simulink model "blocks"  (R2024a)
settings: Solver=VariableStepAuto  StartTime=0.0  StopTime=100000  RelTol=1e-3  AbsTol=1e-3  EnableMultiTasking=on
PreLoadFcn:
  | LeadAcidBatteryWithDashboardBlocksINI;
values from neighbouring files (symbols this model uses):
  Kt = [0.80,1.10,1.20,1.12;]    [LeadAcidBatteryWithDashboardBlocksINI.m]
  Kt_Temps = [25 40 60 75]    [LeadAcidBatteryWithDashboardBlocksINI.m]
  theta_f = -40    [LeadAcidBatteryWithDashboardBlocksINI.m]
  theta_init = 25    [LeadAcidBatteryWithDashboardBlocksINI.m]
libraries: fl_lib x13, nesl_utility x7, LeadAcidBattery_lib x6, SignalEditorBlockLib x1
CloseFcn:
  | try,close(h1_LeadAcidBatteryWithDashboardBlocks),end
  | clear h1_LeadAcidBatteryWithDashboardBlocks
  | 
  | clear simlog_LeadAcidBatteryWithDashboardBlocks
Description:
  | Lead-Acid Battery with Dashboard Blocks
settings Model: PacingRate=2000  Creator=The MathWorks, Inc.  LastModifiedBy=owner's
settings SolverCC: AutoScaleAbsTol=off  AlgebraicLoopSolver=TrustRegion  MaxZcPerStep=1
settings DataIOCC: LimitDataPoints=on  MaxDataPoints=10000  SaveFormat=Array  ReturnWorkspaceOutputs=off
settings OptimizationCC: ReuseModelBlockBuffer=off  LifeSpan=inf
settings DebuggingCC: UnconnectedInputMsg=warning  UnconnectedOutputMsg=warning  UnconnectedLineMsg=warning  AllowSymbolicDim=off  PregeneratedLibrarySubsystemCodeDiagnostic=none  SFUnexpectedBacktrackingDiag=warning  SFNoUnconditionalDefaultTransitionDiag=warning  SFExecutionAtInitializationDiag=none  ArithmeticOperatorsInVariantConditions=warning
settings HardwareCC: ProdBitPerPointer=32  ProdBitPerSizeT=32  ProdBitPerPtrDiffT=32  ProdLargestAtomicFloat=None  ProdIntDivRoundTo=Undefined  ProdEndianess=Unspecified  ProdWordSize=32  ProdHWDeviceType=32-bit Generic
settings ModelReferenceCC: EnableRefExpFcnMdlSchedulingChecks=on  PropagateSignalLabelsOutOfModel=off
settings SFSimCC: SimUseLocalCustomCode=off  CustomCodeUndefinedFunction=UseInterfaceOnly
settings RTWCC: RTWUseLocalCustomCode=off  GPUComputeCapability=3.5  DLArmComputeVersion=19.05
settings CodeAppCC: StateflowObjectComments=on
settings GRTTargetCC: TargetLangStandard=C89/C90 (ANSI)
settings ConfigComp: CovMetricSettings=dw  CovSaveCumulativeToWorkspaceVar=on  CovSaveSingleToWorkspaceVar=on  CovExternalEMLEnable=off  CovSFcnEnable=off
settings SimscapeCC: SimscapeLogType=all  SimscapeLogSimulationStatistics=on  SimscapeLogToSDI=on  SimscapeLogName=simlog_LeadAcidBatteryWithDashboardBlocks  SimscapeLogDataHistory=10000

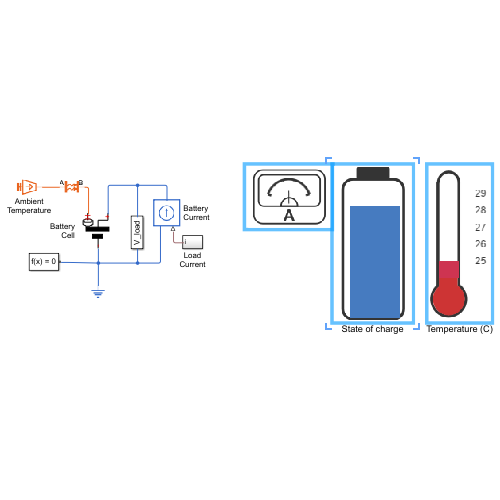
[thumbnail: Simulink's stored preview of the top-level diagram]
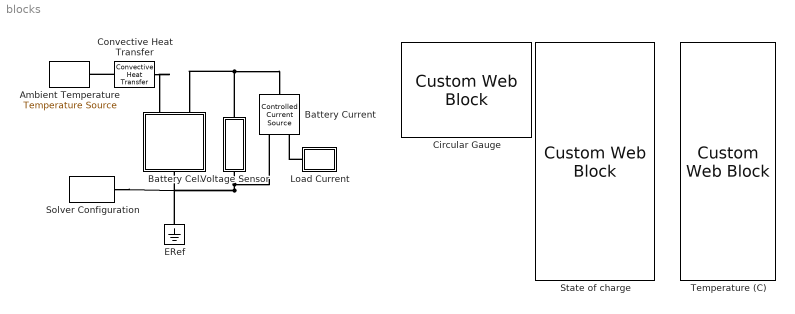
== system blocks ==
  Ambient Temperature : fl_lib/Thermal/Thermal Sources/Temperature Source  temperature=25 degC
  Battery Cell : Subsystem  Tag=PublishSubsystem
      mask Display:
      | % Battery icon
      | plot([0 0],[-1.5 -0.4])
      | plot([0 0 0.8 0.8],[0.2 0.9 0.9 1.5])
      | patch([-1 1 1 -1]*0.4,[1 1 -1 -1]*0.15-0.5,[0;0;0]);
      | patch([-1 1 1 -1]*0.9,[1 1 -1 -1]*0.15+0.1,[0;0;0]);
      | 
      | % Thermal port
      | plot([-1.2,-1.2],[0.5,0.9])
      | plot([-0.4,-0.4],[0.5,0.9])
      | plot([-0.8,-0.8],[0.9,1.5])
      | plot(0.35*cos(0:2*pi/50:2*pi)-0.8,0.15*sin(0:2*pi/50:2*pi)+0.85)
      | plot(0.35*cos(pi:2*pi/50:2*pi)-0.8,0.15*sin(pi:2*pi/50:2*pi)+0.55)
      | 
      | % Plot points to set plot range
      | color('white');plot(1.5,1.5);plot(-1.5,-1.5)
      | 
      | color('red')
      | port_label('LConn',1,'H')
      | port_label('LConn',2,'+')
      | port_label('RConn',1,'-')
  Battery Current : fl_lib/Electrical/Electrical Sources/Controlled Current Source
  Circular Gauge : CustomWebBlock  LabelPosition=Hide  ShowInitialText=on  Configuration="{\"components\":[{\"name\":\"CircularScaleComponent\",\"settings\":{\"bounds\":{\"max\":12,\"min\":-12,\"tickInterval\":23.9999999999999},\"direction\":\"cw\",\"flipLimits\":0,\"innerRadius\":0.75,\"internalTickHeightScaleFactor\":1,\"labelColor\":[38,38,38],\"labelFont\":{\"font\":\"Arial\",\"fontSize\":12},\"labelRadius\":0.528,\"labelTransparency\":0,\"minorTickHeightScaleFactor\":0.2,\"needleImage\":{\"size\":[96,288],\"src\":\"data:image\\/svg+xml;base64,PHN2ZyB3aWR0aD0iOTYiIGhlaWdodD0iMjg4IiB4bWxucz0iaHR0cDovL3d3dy53My5vcmcvMjAwMC9zdmciIHhtbG5zOnhsaW5rPSJodHRwOi8vd3d3LnczLm9yZy8xOTk5L3hsaW5rIiBvdmVyZmxvdz0iaGlkZGVuIj48ZGVmcz48Y2xpcFBhdGggaWQ9ImNsaXAwIj48cGF0aCBkPSJNMCAwIDk2IDAgOTYgMjg4IDAgMjg4WiIgZmlsbC1ydWxlPSJldmVub2RkIiBjbGlwLXJ1bGU9ImV2ZW5vZGQiLz48L2NsaXBQYXRoPjwvZGVmcz48ZyBjbGlwLXBhdGg9InVybCgjY2xpcDApIj48cmVjdCB4PSIwIiB5PSIwIiB3aWR0aD0iOTYiIGhlaWdodD0iMjg4IiBmaWxsPSIjRkZGRkZGIiBmaWxsLW9wYWNpdHk9IjAiLz48cGF0aCBkPSJNNDguNTAwMSA0MS41MDAxIDQ4LjUwMDIgMjQ3LjUiIHN0cm9rZT0iIzAwMDAwMCIgc3Ryb2tlLXdpZHRoPSI3IiBzdHJva2UtbGluZWNhcD0icm91bmQiIHN0cm9rZS1taXRlcmxpbWl0PSI4IiBmaWxsPSJub25lIiBmaWxsLXJ1bGU9ImV2ZW5vZGQiLz48L2c+PC9zdmc+\"},\"needleOffset\":[0.09442302068368028,0],\"needleOrientation\":-45,\"needleRotation\":90,\"needleSize\":{\"height\":0.36796446559573437,\"width\":0.26380868795837903},\"outerRadius\":0.9,\"position\":[0.17317708333333334,0.05625,0.891796875,0.7701822916666666],\"referencePoint\":\"auto\",\"scaleAngle\":145.25613527122786,\"scaleAngleOffset\":197.0817568691423,\"scaleColors\":[],\"scaleColorsSize\":0.2,\"scaleDirection\":\"CW\",\"scalePosition\":[0,0,1,1],\"showLabels\":1,\"showMinorTicks\":1,\"showSpanLine\":1,\"showTicks\":1,\"tickColor\":[0,0,0],\"tickTransparency\":1,\"valueBarColor\":[0,114,189],\"valueBarPosition\":[0,0,1,1],\"valueBarSize\":0.2,\"valueBarTransparency\":0}},{\"name\":\"BackgroundImageComponent\",\"settings\":{\"image\":{\"size\":[384,288],\"src\":\"data:image\\/svg+xml;base64,PHN2ZyB3aWR0aD0iMzg0IiBoZWlnaHQ9IjI4OCIgeG1sbnM9Imh0dHA6Ly93d3cudzMub3JnLzIwMDAvc3ZnIiB4bWxuczp4bGluaz0iaHR0cDovL3d3dy53My5vcmcvMTk5OS94bGluayIgb3ZlcmZsb3c9ImhpZGRlbiI+PGRlZnM+PGNsaXBQYXRoIGlkPSJjbGlwMCI+PHBhdGggZD0iTTAgMCAzODQgMCAzODQgMjg4IDAgMjg4WiIgZmlsbC1ydWxlPSJldmVub2RkIiBjbGlwLXJ1bGU9ImV2ZW5vZGQiLz48L2NsaXBQYXRoPjwvZGVmcz48ZyBjbGlwLXBhdGg9InVybCgjY2xpcDApIj48cmVjdCB4PSIwIiB5PSIwIiB3aWR0aD0iMzg0IiBoZWlnaHQ9IjI4OCIgZmlsbD0iI0ZGRkZGRiIvPjxwYXRoIGQ9Ik0yNy41MDAxIDYxLjgzNDJDMjcuNTAwMSAzOS4wMDYgNDYuMDA2IDIwLjUwMDEgNjguODM0MSAyMC41MDAxTDMxNi4xNjYgMjAuNTAwMUMzMzguOTk0IDIwLjUwMDEgMzU3LjUgMzkuMDA2IDM1Ny41IDYxLjgzNDJMMzU3LjUgMjI3LjE2NkMzNTcuNSAyNDkuOTk0IDMzOC45OTQgMjY4LjUgMzE2LjE2NiAyNjguNUw2OC44MzQxIDI2OC41QzQ2LjAwNiAyNjguNSAyNy41MDAxIDI0OS45OTQgMjcuNTAwMSAyMjcuMTY2WiIgc3Ryb2tlPSIjMDAwMDAwIiBzdHJva2Utd2lkdGg9IjciIHN0cm9rZS1taXRlcmxpbWl0PSI4IiBmaWxsPSJub25lIiBmaWxsLXJ1bGU9ImV2ZW5vZGQiLz48dGV4dCBmb250LWZhbWlseT0iQXJpYWwgUm91bmRlZCBNVCxBcmlhbCBSb3VuZGVkIE1UX01TRm9udFNlcnZpY2Usc2Fucy1zZXJpZiIgZm9udC13ZWlnaHQ9IjcwMCIgZm9udC1zaXplPSI3MiIgdHJhbnNmb3JtPSJ0cmFuc2xhdGUoMTY1LjU4MyAyNTQpIj5BPC90ZXh0PjxwYXRoIGQ9Ik00OS41MDAxIDY2LjY2NzFDNDkuNTAwMSA1My4zMiA2MC4zMiA0Mi41MDAxIDczLjY2NzEgNDIuNTAwMUwzMTEuMzMzIDQyLjUwMDFDMzI0LjY4IDQyLjUwMDEgMzM1LjUgNTMuMzIgMzM1LjUgNjYuNjY3MUwzMzUuNSAxNjMuMzMzQzMzNS41IDE3Ni42OCAzMjQuNjggMTg3LjUgMzExLjMzMyAxODcuNUw3My42NjcxIDE4Ny41QzYwLjMyIDE4Ny41IDQ5LjUwMDEgMTc2LjY4IDQ5LjUwMDEgMTYzLjMzM1oiIHN0cm9rZT0iIzAwMDAwMCIgc3Ryb2tlLXdpZHRoPSI3IiBzdHJva2UtbWl0ZXJsaW1pdD0iOCIgZmlsbD0ibm9uZSIgZmlsbC1ydWxlPSJldmVub2RkIi8+PHBhdGggZD0iTTE1My41IDE4N0MxNTMuNSAxNjUuNzM3IDE3MC43MzcgMTQ4LjUgMTkyIDE0OC41IDIxMy4yNjMgMTQ4LjUgMjMwLjUgMTY1LjczNyAyMzAuNSAxODcgMjMwLjUgMTg3LjExNSAyMzAuNSAxODcuMjMgMjMwLjQ5OCAxODcuMzQ2TDE5MiAxODdaIiBzdHJva2U9IiMwMDAwMDAiIHN0cm9rZS13aWR0aD0iNyIgc3Ryb2tlLW1pdGVybGltaXQ9IjgiIGZpbGw9Im5vbmUiIGZpbGwtcnVsZT0iZXZlbm9kZCIvPjwvZz48L3N2Zz4=\",\"srcOrientation\":\"horizontal\"},\"position\":[0,0,1,1],\"scaleMode\":\"0\"}},{\"name\":\"ForegroundImageComponent\",\"settings\":{\"image\":{\"size\":[0,0],\"src\":\"default\",\"srcOrientation\":[]},\"isForeground\":1,\"position\":[0,0,1,1],\"scaleMode\":\"0\"}}],\"settings\":{\"BindingType\":\"signal\",\"aspectRatio\":1.3333333333333333,\"backgroundOffset\":1,\"direction\":\"cw\",\"fixedAspectRatio\":\"on\",\"flipLimits\":0,\"orientation\":\"horizontal\",\"version\":\"R2023a\"},\"type\":\"CircularGauge\"}"
  Convective Heat Transfer : fl_lib/Thermal/Thermal Elements/Convective Heat Transfer  thermal_type=foundation.enum.constant_variable.constant  area=Area m^2  heat_tr_coeff=Rtheta W/(m^2 * K)  min_heat_tr_coeff=1e-3 W/(K*m^2)  T_specify=off  T_priority=None  T=0 K  T_nominal_specify=off  T_nominal_value=1  T_nominal_unit=K  Q_specify=off  Q_priority=None  Q=0 W  Q_nominal_specify=off  Q_nominal_value=1  Q_nominal_unit=W
  ERef : fl_lib/Electrical/Electrical Elements/Electrical Reference
  Load Current : Subsystem
  Solver Configuration : nesl_utility/Solver Configuration  PhysicalDomain=network_engine_domain  SubClassName=solver  LeftPortType=input  RightPortType=generic  Tones=[]  Harmonics=[]  SimulateNoise=off  Profile=off  UseLocalSampling=off  EnableSwitchedLinearOptims=on  FrequencyDomain=off  UseCCode=off  RelTol=0.001  AbsTol=1e-06  MinStep=1e-09  ToWorkspace=off  RevertToSquareIcSolve=off  NumHomotopyIterations=100  PhasorMode=off  PhasorModeNumHarmonics=1  ConsistencySolver=NEWTON_XTOL_AFTER_FTOL  IndexReductionMethod=DerivativeReplacement  DoDC=off  ResidualTolerance=1e-9  ConsistencyTolSource=GLOBAL  ConsistencyAbsTol=0.001  ConsistencyRelTol=0.001  ConsistencyTolFactor=0.001  UseLocalSolver=off  LocalSolverChoice=NE_BACKWARD_EULER_ADVANCER  ResolveIndetEquations=on  FunctionEvalNumThread=1  LocalSolverSampleTime=1  DoFixedCost=off  MaxNonlinIter=3  MaxModeIter=2  ComputeImpulses=off  ImpulseIterations=2  LinearAlgebra=auto  LinearAlgebraNumThread=0  EquationFormulation=NE_TIME_EF  DelaysMemoryBudget=1024  AutomaticFiltering=on  FilteringTimeConstant=0.001  PartitionStorageMethod=AS_NEEDED  PartitionMemoryBudget=1024  PartitionMethod=FAST  MultibodyUseLocalSolver=off  MultibodyLocalSolverChoice=ODE1  MultibodyLocalSolverSampleTime=0.001
  State of charge : CustomWebBlock  LabelPosition=Hide  ShowInitialText=on  Configuration="{\"components\":[{\"name\":\"LinearScaleComponent\",\"settings\":{\"bounds\":{\"max\":1,\"min\":0,\"tickInterval\":0.2},\"internalTickHeightScaleFactor\":0.5,\"labelColor\":[0,0,0],\"labelFont\":{\"font\":\"Arial\",\"fontSize\":12},\"labelOffset\":0.05,\"labelTransparency\":0,\"needleImage\":{\"size\":[0,0],\"src\":\"\",\"srcOrientation\":\"Right\"},\"needleOffset\":[0,0],\"needleSize\":{\"height\":0,\"width\":0},\"position\":[0.0662421218487395,0.10333508403361344,2.7942489495798317,0.9641544117647058],\"referencePoint\":\"auto\",\"scaleColors\":[],\"scaleColorsSize\":0.2,\"scaleDirection\":\"BT\",\"showLabels\":1,\"showMinorTicks\":0,\"showSpanLine\":1,\"showTicks\":1,\"tickColor\":[38,38,38],\"tickTransparency\":0,\"valueBarColor\":[23,89,176],\"valueBarOffset\":0,\"valueBarSize\":0.23,\"valueBarTransparency\":1}},{\"name\":\"BackgroundImageComponent\",\"settings\":{\"image\":{\"size\":[192,384],\"src\":\"data:image\\/svg+xml;base64,PHN2ZyB3aWR0aD0iMTkyIiBoZWlnaHQ9IjM4NCIgeG1sbnM9Imh0dHA6Ly93d3cudzMub3JnLzIwMDAvc3ZnIiB4bWxuczp4bGluaz0iaHR0cDovL3d3dy53My5vcmcvMTk5OS94bGluayIgb3ZlcmZsb3c9ImhpZGRlbiI+PGRlZnM+PGNsaXBQYXRoIGlkPSJjbGlwMCI+PHBhdGggZD0iTTAgMCAxOTIgMCAxOTIgMzg0IDAgMzg0WiIgZmlsbC1ydWxlPSJldmVub2RkIiBjbGlwLXJ1bGU9ImV2ZW5vZGQiLz48L2NsaXBQYXRoPjwvZGVmcz48ZyBjbGlwLXBhdGg9InVybCgjY2xpcDApIj48cmVjdCB4PSIwIiB5PSIwIiB3aWR0aD0iMTkyIiBoZWlnaHQ9IjM4NCIgZmlsbD0iI0ZGRkZGRiIvPjxwYXRoIGQ9Ik0yMi41MDAxIDU4LjUwMDVDMjIuNTAwMSA0NC42OTMxIDMzLjY5MzEgMzMuNTAwMSA0Ny41MDA1IDMzLjUwMDFMMTQ3LjUgMzMuNTAwMUMxNjEuMzA3IDMzLjUwMDEgMTcyLjUgNDQuNjkzMSAxNzIuNSA1OC41MDA1TDE3Mi41IDM1My41QzE3Mi41IDM2Ny4zMDcgMTYxLjMwNyAzNzguNSAxNDcuNSAzNzguNUw0Ny41MDA1IDM3OC41QzMzLjY5MzEgMzc4LjUgMjIuNTAwMSAzNjcuMzA3IDIyLjUwMDEgMzUzLjVaIiBzdHJva2U9IiMwMDAwMDAiIHN0cm9rZS13aWR0aD0iNyIgc3Ryb2tlLW1pdGVybGltaXQ9IjgiIGZpbGw9Im5vbmUiIGZpbGwtcnVsZT0iZXZlbm9kZCIvPjxwYXRoIGQ9Ik01NiA4LjAwMDA5QzU2IDUuMjM4NjIgNTguMjM4NiAzIDYxLjAwMDEgM0wxMzMgM0MxMzUuNzYxIDMgMTM4IDUuMjM4NjIgMTM4IDguMDAwMDlMMTM4IDI3Ljk5OTlDMTM4IDMwLjc2MTQgMTM1Ljc2MSAzMyAxMzMgMzNMNjEuMDAwMSAzM0M1OC4yMzg2IDMzIDU2IDMwLjc2MTQgNTYgMjcuOTk5OVoiIGZpbGwtcnVsZT0iZXZlbm9kZCIvPjwvZz48L3N2Zz4=\",\"srcOrientation\":\"vertical\"},\"position\":[0,0,1,1],\"scaleMode\":\"0\"}},{\"name\":\"ForegroundImageComponent\",\"settings\":{\"image\":{\"size\":[0,0],\"src\":\"default\",\"srcOrientation\":[]},\"isForeground\":1,\"position\":[0,0,1,1],\"scaleMode\":\"0\"}}],\"settings\":{\"BindingType\":\"signal\",\"aspectRatio\":0.5,\"backgroundColor\":[0,0,0],\"backgroundOffset\":0,\"backgroundOpacity\":1,\"fixedAspectRatio\":\"on\",\"orientation\":\"vertical\",\"showBackgroundColor\":0,\"version\":\"R2023a\"},\"type\":\"LinearGauge\"}"
  Temperature (C) : CustomWebBlock  LabelPosition=Hide  ShowInitialText=on  Configuration="{\"components\":[{\"name\":\"LinearScaleComponent\",\"settings\":{\"bounds\":{\"max\":30,\"min\":24,\"tickInterval\":\"auto\"},\"internalTickHeightScaleFactor\":0.5,\"labelColor\":[0,0,0],\"labelFont\":{\"font\":\"Arial\",\"fontSize\":12},\"labelOffset\":0.05,\"labelTransparency\":1,\"needleImage\":{\"size\":[0,0],\"src\":\"\",\"srcOrientation\":\"Right\"},\"needleOffset\":[0,0],\"needleSize\":{\"height\":0,\"width\":0},\"position\":[0.028426995798319327,0.0802226588081205,1.3551080550098231,0.7288602941176471],\"referencePoint\":\"auto\",\"scaleColors\":[],\"scaleColorsSize\":0.2,\"scaleDirection\":\"BT\",\"showLabels\":1,\"showMinorTicks\":0,\"showSpanLine\":1,\"showTicks\":1,\"tickColor\":[250,245,200],\"tickTransparency\":0,\"valueBarColor\":[194,0,36],\"valueBarOffset\":0,\"valueBarSize\":0.23,\"valueBarTransparency\":1}},{\"name\":\"BackgroundImageComponent\",\"settings\":{\"image\":{\"size\":[154,384],\"src\":\"data:image\\/svg+xml;base64,PHN2ZyB3aWR0aD0iMTU0IiBoZWlnaHQ9IjM4NCIgeG1sbnM9Imh0dHA6Ly93d3cudzMub3JnLzIwMDAvc3ZnIiB4bWxuczp4bGluaz0iaHR0cDovL3d3dy53My5vcmcvMTk5OS94bGluayIgb3ZlcmZsb3c9ImhpZGRlbiI+PGRlZnM+PGNsaXBQYXRoIGlkPSJjbGlwMCI+PHBhdGggZD0iTTAgMCAxNTQgMCAxNTQgMzg0IDAgMzg0WiIgZmlsbC1ydWxlPSJldmVub2RkIiBjbGlwLXJ1bGU9ImV2ZW5vZGQiLz48L2NsaXBQYXRoPjwvZGVmcz48ZyBjbGlwLXBhdGg9InVybCgjY2xpcDApIj48cmVjdCB4PSIwIiB5PSIwIiB3aWR0aD0i ...(+1892 chars)\",\"srcOrientation\":\"vertical\"},\"position\":[0,0,1,1],\"scaleMode\":\"0\"}},{\"name\":\"ForegroundImageComponent\",\"settings\":{\"image\":{\"size\":[0,0],\"src\":\"default\",\"srcOrientation\":[]},\"isForeground\":1,\"position\":[0,0,1,1],\"scaleMode\":\"0\"}}],\"settings\":{\"BindingType\":\"signal\",\"aspectRatio\":0.4010416666666667,\"backgroundColor\":[0,0,0],\"backgroundOffset\":0,\"backgroundOpacity\":1,\"fixedAspectRatio\":\"on\",\"orientation\":\"vertical\",\"showBackgroundColor\":0,\"version\":\"R2023a\"},\"type\":\"LinearGauge\"}"
  Voltage Sensor : Subsystem
      mask Display: disp('V_load')
  connections:
  Voltage Sensor/RConn1 -- Battery Current/RConn2 -- ERef/LConn1 -- Solver Configuration/RConn1 -- Battery Cell/RConn1
  Voltage Sensor/LConn1 -- Battery Cell/LConn2 -- Battery Current/LConn1
  Convective Heat Transfer/RConn1 -- Battery Cell/LConn1
  Convective Heat Transfer/LConn1 -- Ambient Temperature/LConn1
  Load Current/RConn1 -- Battery Current/RConn1

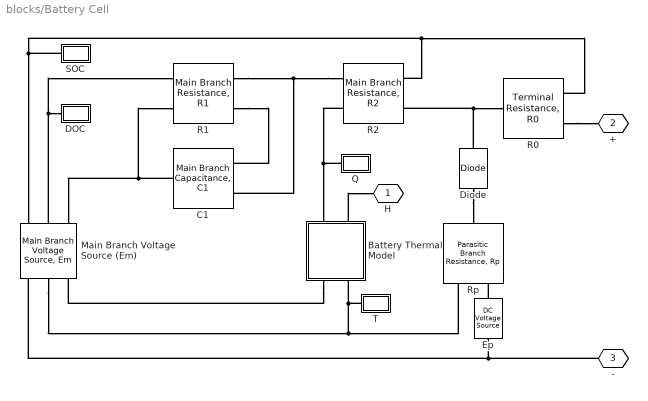
== system blocks/Battery Cell ==
  " DOC " : Subsystem
  " SOC " : Subsystem
  Battery Thermal Model : Subsystem  Tag=PublishSubsystem
  C1 : LeadAcidBattery_lib/Main Branch Capacitance, C1  Tau1=Tau1 s  Cmin=1e-5 F
      settings: InternalSimscapePortConfiguration="{\"Bottom\":[],\"Left\":[{\"id\":\"R1\",\"label\":\"R1\",\"type\":\"input\"},{\"id\":\"p\",\"label\":\"+\",\"type\":\"foundation.electrical.electrical\"}],\"Right\":[{\"id\":\"n\",\"label\":\"-\",\"type\":\"foundation.electrical.electrical\"}],\"Top\":[]}"
  Diode : fl_lib/Electrical/Electrical Elements/Diode  Vf=0.6 V  Ron=0.3 Ohm  Goff=1e-5 1/Ohm  i_specify=off  i_priority=High  i=0 A  i_nominal_specify=off  i_nominal_value=1  i_nominal_unit=A  v_specify=off  v_priority=High  v=0 V  v_nominal_specify=off  v_nominal_value=1  v_nominal_unit=V
  Ep : fl_lib/Electrical/Electrical Sources/DC Voltage Source  v0=Ep V
  Main Branch Voltage Source (Em) : LeadAcidBattery_lib/Main Branch Voltage Source, Em  Em0=Emo V  Ke=Ke V/K  Kc=Kc  C0=Costar s*A  Istar=Istar A  delta=delta  Tau1=Tau1 s  Qinit=Qe_init s*A
      settings: InternalSimscapePortConfiguration="{\"Bottom\":[],\"Left\":[{\"id\":\"SOC\",\"label\":\"SOC\",\"type\":\"output\"},{\"id\":\"DOC\",\"label\":\"DOC\",\"type\":\"output\"},{\"id\":\"p\",\"label\":\"+\",\"type\":\"foundation.electrical.electrical\"}],\"Right\":[{\"id\":\"n\",\"label\":\"-\",\"type\":\"foundation.electrical.electrical\"},{\"id\":\"T\",\"label\":\"T\",\"type\":\"input\"},{\"id\":\"Kt\",\"label\":\"Kt\",\"type\":\"input\"}],\"Top\":[]}"
  Q : Subsystem
  R0 : LeadAcidBattery_lib/Terminal Resistance, R0  R00=Roo Ohm  A0=Ao
      settings: InternalSimscapePortConfiguration="{\"Bottom\":[],\"Left\":[{\"id\":\"SOC\",\"label\":\"SOC\",\"type\":\"input\"},{\"id\":\"p\",\"label\":\"+\",\"type\":\"foundation.electrical.electrical\"}],\"Right\":[{\"id\":\"n\",\"label\":\"-\",\"type\":\"foundation.electrical.electrical\"}],\"Top\":[]}"
  R1 : LeadAcidBattery_lib/Main Branch Resistance, R1  R10=R10 Ohm  DOC_min=1e-006
      settings: InternalSimscapePortConfiguration="{\"Bottom\":[],\"Left\":[{\"id\":\"p\",\"label\":\"+\",\"type\":\"foundation.electrical.electrical\"},{\"id\":\"R1\",\"label\":\"R1\",\"type\":\"output\"}],\"Right\":[{\"id\":\"DOC\",\"label\":\"DOC\",\"type\":\"input\"},{\"id\":\"n\",\"label\":\"-\",\"type\":\"foundation.electrical.electrical\"}],\"Top\":[]}"
  R2 : LeadAcidBattery_lib/Main Branch Resistance, R2  R20=R20 Ohm  A21=A21  A22=A22  Istar=Istar A
      settings: InternalSimscapePortConfiguration="{\"Bottom\":[],\"Left\":[{\"id\":\"SOC\",\"label\":\"SOC\",\"type\":\"input\"},{\"id\":\"p\",\"label\":\"+\",\"type\":\"foundation.electrical.electrical\"}],\"Right\":[{\"id\":\"n\",\"label\":\"-\",\"type\":\"foundation.electrical.electrical\"},{\"id\":\"pow\",\"label\":\"POW\",\"type\":\"output\"}],\"Top\":[]}"
  Rp : LeadAcidBattery_lib/Parasitic Branch Resistance, Rp  Gp0=Gpo 1/Ohm  Vp0=Vpo V  Ap=Ap  Tf=theta_f degC
      settings: InternalSimscapePortConfiguration="{\"Bottom\":[],\"Left\":[{\"id\":\"p\",\"label\":\"+\",\"type\":\"foundation.electrical.electrical\"}],\"Right\":[{\"id\":\"theta\",\"label\":\"T\",\"type\":\"input\"},{\"id\":\"n\",\"label\":\"-\",\"type\":\"foundation.electrical.electrical\"}],\"Top\":[]}"
  T : Subsystem
  H : PMIOPort  Tag=PMCPort  Side=Left
  + : PMIOPort  Tag=PMCPort  Port=2  Side=Left
  - : PMIOPort  Tag=PMCPort  Port=3  Side=Right
  connections:
  Battery Thermal Model/RConn2 -- T/LConn1 -- Rp/RConn1 -- Main Branch Voltage Source (Em)/RConn2
  R0/LConn2 -- +/RConn1
  " DOC "/LConn1 -- R1/RConn1 -- Main Branch Voltage Source (Em)/LConn2
  C1/RConn1 -- R1/RConn2 -- Main Branch Voltage Source (Em)/LConn3
  R2/RConn1 -- C1/LConn2 -- R1/LConn1
  R1/LConn2 -- C1/LConn1
  R0/LConn1 -- " SOC "/LConn1 -- Main Branch Voltage Source (Em)/LConn1 -- R2/LConn1
  Battery Thermal Model/LConn2 -- H/RConn1
  Ep/LConn1 -- Rp/RConn2
  Diode/RConn1 -- Rp/LConn1
  Battery Thermal Model/RConn1 -- Main Branch Voltage Source (Em)/RConn3
  Ep/RConn1 -- Main Branch Voltage Source (Em)/RConn1 -- -/RConn1
  R2/RConn2 -- Q/LConn1 -- Battery Thermal Model/LConn1
  R2/LConn2 -- R0/RConn1 -- Diode/LConn1

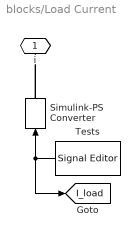
== system blocks/Load Current ==
  Simulink-PS Converter : nesl_utility/Simulink-PS Converter  PhysicalDomain=network_engine_domain  SubClassName=ps_input  LeftPortType=input  RightPortType=output  PseudoPeriodic=off  Frequencies=[]  NoiseDistribution=none  NoiseParameters=[]  Unit=A  AffineConversion=off  FilteringAndDerivatives=zero  SimscapeFilterOrder=1  InputFilterTimeConstant=.001  UdotUserProvided=0
  Tests : SignalEditorBlockLib/Signal Editor  FileName=LeadAcidBatteryWithDashboardBlocksLoadCurrentTests.mat  ActiveScenario=Charge_Cycle  ActiveSignal=Current  IsBus=off  OutputBusObjectStr=Bus: BusObject  SampleTime=0  OutputAfterFinalValue=Extrapolation  Unit=inherit  PreserveSignalName=on  ApplySigPropsToAllScenarios=on  ApplySigPropsToAllSignals=off
  i : PMIOPort  Side=Right
  tag scope: I_load=global
  wires:
  Tests/1 -> Simulink-PS Converter/1, [I_load]
  connections:
  Simulink-PS Converter/RConn1 -- i/RConn1

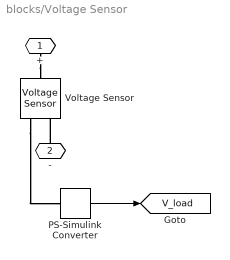
== system blocks/Voltage Sensor ==
  PS-Simulink Converter : nesl_utility/PS-Simulink Converter  PhysicalDomain=network_engine_domain  SubClassName=ps_output  LeftPortType=input  RightPortType=output  PseudoPeriodic=off  Frequencies=[]  VectorFormat=1-D array  Unit=V  AffineConversion=off
  Voltage Sensor : fl_lib/Electrical/Electrical Sensors/Voltage Sensor
  + : PMIOPort  Side=Left
  - : PMIOPort  Port=2  Side=Right
  tag scope: V_load=global
  wires:
  PS-Simulink Converter/1 -> [V_load]
  connections:
  Voltage Sensor/RConn1 -- PS-Simulink Converter/LConn1
  +/RConn1 -- Voltage Sensor/LConn1
  -/RConn1 -- Voltage Sensor/RConn2

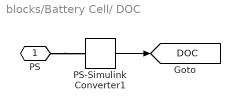
== system blocks/Battery Cell/ DOC  ==
  PS-Simulink Converter1 : nesl_utility/PS-Simulink Converter  PhysicalDomain=network_engine_domain  SubClassName=ps_output  LeftPortType=input  RightPortType=output  PseudoPeriodic=off  Frequencies=[]  VectorFormat=1-D array  Unit=1  AffineConversion=off
  PS : PMIOPort  Side=Left
  tag scope: DOC=global
  wires:
  PS-Simulink Converter1/1 -> [DOC]
  connections:
  PS/RConn1 -- PS-Simulink Converter1/LConn1

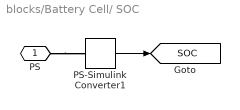
== system blocks/Battery Cell/ SOC  ==
  PS-Simulink Converter1 : nesl_utility/PS-Simulink Converter  PhysicalDomain=network_engine_domain  SubClassName=ps_output  LeftPortType=input  RightPortType=output  PseudoPeriodic=off  Frequencies=[]  VectorFormat=1-D array  Unit=1  AffineConversion=off
  PS : PMIOPort  Side=Left
  tag scope: SOC=global
  wires:
  PS-Simulink Converter1/1 -> [SOC]
  connections:
  PS/RConn1 -- PS-Simulink Converter1/LConn1

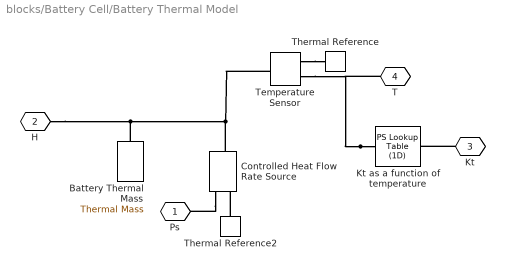
== system blocks/Battery Cell/Battery Thermal Model ==
  Battery Thermal Mass : fl_lib/Thermal/Thermal Elements/Thermal Mass  mass_type=foundation.enum.constant_variable.constant  mass=1 kg  sp_heat=Ctheta J/kg/K  mass_min=1e-6 kg  num_ports=foundation.enum.numPorts2.one  m_specify=off  m_priority=High  m=1 kg  m_nominal_specify=off  m_nominal_value=1  m_nominal_unit=kg  T_specify=on  T_priority=High  T=theta_init degC  T_nominal_specify=off  T_nominal_value=1  T_nominal_unit=K  Q_specify=off  Q_priority=None  Q=0 W  Q_nominal_specify=off  Q_nominal_value=1  Q_nominal_unit=W
  Controlled Heat Flow Rate Source : fl_lib/Thermal/Thermal Sources/Controlled Heat Flow Rate Source
  Kt as a function of temperature : fl_lib/Physical Signals/Lookup Tables/PS Lookup Table (1D)  x=[theta_f, Kt_Temps]+273 K  f=[0 Kt]  interp_method=simscape.enum.interpolation.linear  extrap_method=simscape.enum.extrapolation.linear
  Temperature Sensor : fl_lib/Thermal/Thermal Sensors/Temperature Sensor  temperature_measure=foundation.enum.MeasurementReference.difference
  Thermal Reference : fl_lib/Thermal/Thermal Elements/Thermal Reference
  Thermal Reference2 : fl_lib/Thermal/Thermal Elements/Thermal Reference
  Ps : PMIOPort  Tag=PMCPort  Side=Left
  H : PMIOPort  Tag=PMCPort  Port=2  Side=Left
  Kt : PMIOPort  Tag=PMCPort  Port=3  Side=Right
  T : PMIOPort  Tag=PMCPort  Port=4  Side=Right
  connections:
  Temperature Sensor/RConn1 -- Thermal Reference/LConn1
  Kt as a function of temperature/LConn1 -- Temperature Sensor/RConn2 -- T/RConn1
  Thermal Reference2/LConn1 -- Controlled Heat Flow Rate Source/RConn2
  H/RConn1 -- Battery Thermal Mass/LConn1 -- Temperature Sensor/LConn1 -- Controlled Heat Flow Rate Source/LConn1
  Kt/RConn1 -- Kt as a function of temperature/RConn1
  Controlled Heat Flow Rate Source/RConn1 -- Ps/RConn1

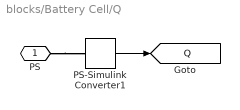
== system blocks/Battery Cell/Q ==
  PS-Simulink Converter1 : nesl_utility/PS-Simulink Converter  PhysicalDomain=network_engine_domain  SubClassName=ps_output  LeftPortType=input  RightPortType=output  PseudoPeriodic=off  Frequencies=[]  VectorFormat=1-D array  Unit=W  AffineConversion=on
  PS : PMIOPort  Side=Left
  tag scope: Q=global
  wires:
  PS-Simulink Converter1/1 -> [Q]
  connections:
  PS/RConn1 -- PS-Simulink Converter1/LConn1

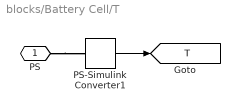
== system blocks/Battery Cell/T ==
  PS-Simulink Converter1 : nesl_utility/PS-Simulink Converter  PhysicalDomain=network_engine_domain  SubClassName=ps_output  LeftPortType=input  RightPortType=output  PseudoPeriodic=off  Frequencies=[]  VectorFormat=1-D array  Unit=degC  AffineConversion=on
  PS : PMIOPort  Side=Left
  tag scope: T=global
  wires:
  PS-Simulink Converter1/1 -> [T]
  connections:
  PS/RConn1 -- PS-Simulink Converter1/LConn1
